simulink model "DYNctl_ver4_etud_lineaire"  (R2014b)
settings: Solver=ode45  StartTime=0.0  StopTime=tfin  FixedStep=0.001  RelTol=1e-09
values from neighbouring files (symbols this model uses):
  A = sym('A', [13 13])    [MatlabProjet.m]    (also in bancessai_ini.m = double(subs(A)); equilibre.m = double(subs(A)))
  B = sym('B', [13 3])    [MatlabProjet.m]    (also in bancessai_ini.m = double(subs(B)); equilibre.m = double(subs(B)))
  C = sym('B', [7 13])    [MatlabProjet.m]    (also in bancessai_ini.m = double(subs(C)); equilibre.m = double(subs(C)); interpolationGenerique.m = phi\y)
  D = zeros(7, 3)    [MatlabProjet.m]    (also in bancessai_ini.m = double(subs(D)); equilibre.m = double(subs(D)); matrices_syms.m)
  v_sx_eq = 0    [MatlabEquilibre.m]
  v_sy_eq = 0    [MatlabEquilibre.m]
  Va_eq = R_bobine * Ia_eq    [MatlabEquilibre.m]    (also in bancessai_ini.m = Ia_eq*R_bobine; equilibre.m = Ia_eq*R_bobine)
  xs_eq = xs    (= 0)    [equilibre.m]
  ys_eq = ys    (= 0)    [equilibre.m]
undefined symbols (not defined in the file or in its folder): sym2poly, zD_eq, zE_eq, zF_eq
settings Model: Creator=delafontaine  LastModifiedBy=Eric
settings SolverCC: AlgebraicLoopSolver=LineSearch
settings DataIOCC: SignalLoggingSaveFormat=ModelDataLogs
settings DebuggingCC: UnderspecifiedInitializationDetection=Classic  MergeDetectMultiDrivingBlocksExec=none  SolverPrmCheckMsg=none  MultiTaskDSMMsg=warning  MultiTaskCondExecSysMsg=none  FrameProcessingCompatibilityMsg=error
settings RTWCC: IncludeERTFirstTime=on

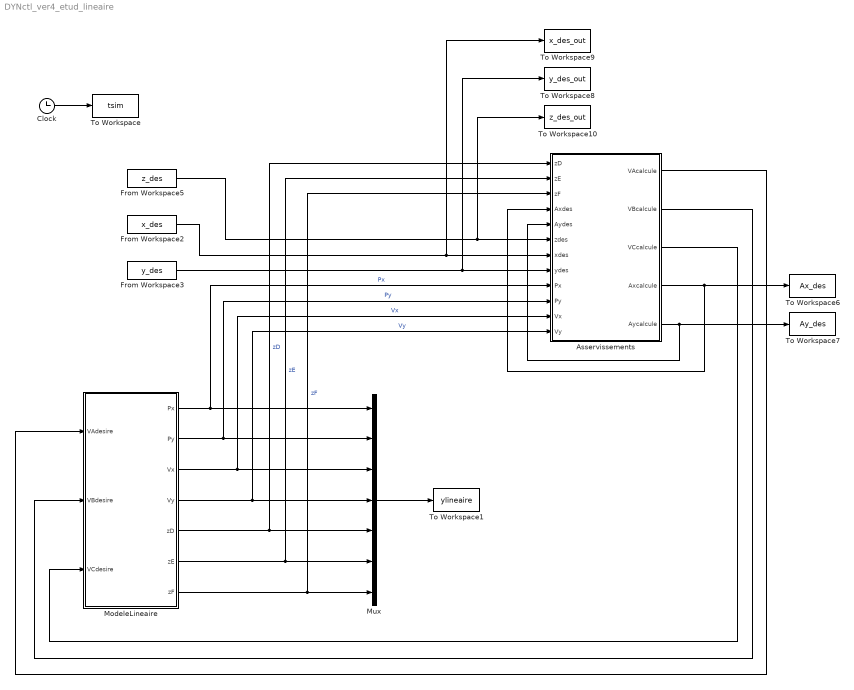
== system DYNctl_ver4_etud_lineaire ==
  Asservissements : Subsystem
      mask help: Simulink:masks:GenSFuncDesc_MD
      mask Help: eval('feval(''rtwprivate'',''rtwhelpview'',''rtw_sfcn_block'')');
  Clock : Clock
  From Workspace2 : FromWorkspace  VariableName=x_des  SampleTime=0  Interpolate=off  OutputAfterFinalValue=Holding final value
  From Workspace3 : FromWorkspace  VariableName=y_des  SampleTime=0  Interpolate=off  OutputAfterFinalValue=Holding final value
  From Workspace5 : FromWorkspace  VariableName=z_des  SampleTime=0  Interpolate=off  OutputAfterFinalValue=Holding final value
  ModeleLineaire : Subsystem
      mask help: Simulink:masks:GenSFuncDesc_MD
      mask Help: eval('feval(''rtwprivate'',''rtwhelpview'',''rtw_sfcn_block'')');
  Mux : Mux  Inputs=7
  To Workspace : ToWorkspace  VariableName=tsim  SampleTime=-1
  To Workspace1 : ToWorkspace  VariableName=ylineaire  SampleTime=-1
  To Workspace10 : ToWorkspace  VariableName=z_des_out  SampleTime=-1
  To Workspace6 : ToWorkspace  VariableName=Ax_des  SampleTime=-1
  To Workspace7 : ToWorkspace  VariableName=Ay_des  SampleTime=-1
  To Workspace8 : ToWorkspace  VariableName=y_des_out  SampleTime=-1
  To Workspace9 : ToWorkspace  VariableName=x_des_out  SampleTime=-1
  wires:
  Clock/1 -> To Workspace/1
  From Workspace5/1 -> To Workspace10/1, Asservissements/6(zdes)
  From Workspace3/1 -> Asservissements/8(ydes), To Workspace8/1
  From Workspace2/1 -> Asservissements/7(xdes), To Workspace9/1
  Asservissements/4(Axcalcule) -> Asservissements/4(Axdes), To Workspace6/1
  Asservissements/5(Aycalcule) -> Asservissements/5(Aydes), To Workspace7/1
  Asservissements/1(VAcalcule) -> ModeleLineaire/1(VAdesire)
  Asservissements/2(VBcalcule) -> ModeleLineaire/2(VBdesire)
  Asservissements/3(VCcalcule) -> ModeleLineaire/3(VCdesire)
  ModeleLineaire/5(zD) -> Mux/5, Asservissements/1(zD)  "zD"
  ModeleLineaire/6(zE) -> Mux/6, Asservissements/2(zE)  "zE"
  ModeleLineaire/7(zF) -> Mux/7, Asservissements/3(zF)  "zF"
  ModeleLineaire/1(Px) -> Mux/1, Asservissements/9(Px)  "Px"
  ModeleLineaire/2(Py) -> Asservissements/10(Py), Mux/2  "Py"
  ModeleLineaire/3(Vx) -> Asservissements/11(Vx), Mux/3  "Vx"
  ModeleLineaire/4(Vy) -> Asservissements/12(Vy), Mux/4  "Vy"
  Mux/1 -> To Workspace1/1

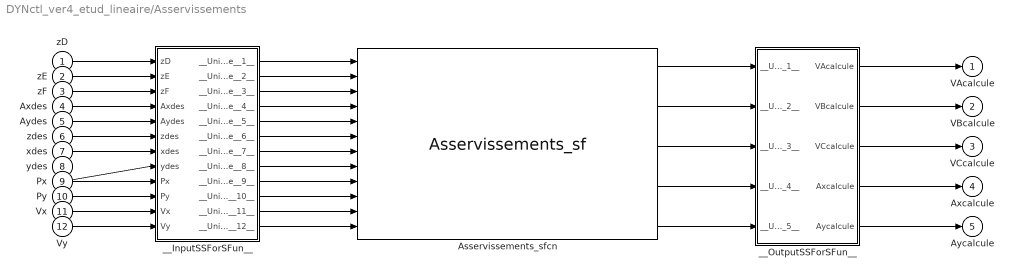
== system DYNctl_ver4_etud_lineaire/Asservissements ==
  zD : Inport
  zE : Inport  Port=2
  zF : Inport  Port=3
  Axdes : Inport  Port=4
  Aydes : Inport  Port=5
  zdes : Inport  Port=6
  xdes : Inport  Port=7
  ydes : Inport  Port=8
  Px : Inport  Port=9
  Py : Inport  Port=10
  Vx : Inport  Port=11
  Vy : Inport  Port=12
  Asservissements_sfcn : S-Function  FunctionName=Asservissements_sf  SFunctionModules=""  EnableBusSupport=off  mask{rtw_sf_name=Asservissements_sf, showVar=off}
      mask prompts: rtw_sf_name "Simulink:masks:GenSFuncName_MP"; showVar "Simulink:masks:GenSFuncShowModuleList_MP"
      mask help: Simulink:masks:GenSFuncDesc_MD
      mask init:
      | displist = '';
      | if ~strcmp(get_param(gcb, 'FunctionName'), rtw_sf_name);
      |   set_param(gcb, 'FunctionName', rtw_sf_name);
      | end
      | % Check if we are generating code
      | rtw_mode = false;
      | if strcmpi(get_param(bdroot(gcb),'SimulationStatus'),'Initializing')
      | 	rtw_mode = strcmpi(get_param(bdroot(gcb),'BuildingRTWCode'),'on') && ...
      | 		~strcmpi(get_param(bdroot(gcb),'TargetStyle'),'SimulationTarget');
      | end
      | if showVar || rtw_mode
      | 	if exist('rtwsfunc') == 2 | exist('rtwsfunc') == 6
      | 		tmplist = rtwsfunc(rtw_sf_name,gcb);
      | 		tmplist = DAStudio.message('Simulink:masks:GenSFuncListOfModules_IC', tmplist);
      | 	elseif showVar
      | 		tmplist1 = DAStudio.message('Simulink:masks:GenSFuncListOfModules_IC', '');
      |         tmplist2 = DAStudio.message('Simulink:masks:GenSFuncNotLicensed_IC');
      |         tmplist = [tmplist1 tmplist2];
      |  	end
      | end
      | if showVar
      |   displist = tmplist;
      | end
      settings: CopyFcn=|
      | if ~strcmp(get_param(gcb,'Linkstatus'),'none') && ...
      | ~strcmp(get_param(gcb,'Linkstatus'),'implicit')
      |   set_param(gcb,'LinkStatus','none');
      | end
      mask Help: eval('feval(''rtwprivate'',''rtwhelpview'',''rtw_sfcn_block'')');
      mask Display:
      | port_label('input',1,'zD');
      | port_label('input',2,'zE');
      | port_label('input',3,'zF');
      | port_label('input',4,'Axdes');
      | port_label('input',5,'Aydes');
      | port_label('input',6,'zdes');
      | port_label('input',7,'xdes');
      | port_label('input',8,'ydes');
      | port_label('input',9,'Px');
      | port_label('input',10,'Py');
      | port_label('input',11,'Vx');
      | port_label('input',12,'Vy');
      | port_label('output',1,'VAcalcule');
      | port_label('output',2,'VBcalcule');
      | port_label('output',3,'VCcalcule');
      | port_label('output',4,'Axcalcule');
      | port_label('output',5,'Aycalcule');
  __InputSSForSFun__ : Subsystem
  __OutputSSForSFun__ : Subsystem
  VAcalcule : Outport
  VBcalcule : Outport  Port=2
  VCcalcule : Outport  Port=3
  Axcalcule : Outport  Port=4
  Aycalcule : Outport  Port=5
  wires:
  zD/1 -> __InputSSForSFun__/1(zD)
  zE/1 -> __InputSSForSFun__/2(zE)
  zF/1 -> __InputSSForSFun__/3(zF)
  Axdes/1 -> __InputSSForSFun__/4(Axdes)
  Aydes/1 -> __InputSSForSFun__/5(Aydes)
  zdes/1 -> __InputSSForSFun__/6(zdes)
  xdes/1 -> __InputSSForSFun__/7(xdes)
  ydes/1 -> __InputSSForSFun__/8(ydes)
  Px/1 -> __InputSSForSFun__/9(Px)
  Py/1 -> __InputSSForSFun__/10(Py)
  Vx/1 -> __InputSSForSFun__/11(Vx)
  Vy/1 -> __InputSSForSFun__/12(Vy)
  __InputSSForSFun__/1(__UniqueOutportName__1__) -> Asservissements_sfcn/1
  __InputSSForSFun__/2(__UniqueOutportName__2__) -> Asservissements_sfcn/2
  __InputSSForSFun__/3(__UniqueOutportName__3__) -> Asservissements_sfcn/3
  __InputSSForSFun__/4(__UniqueOutportName__4__) -> Asservissements_sfcn/4
  __InputSSForSFun__/5(__UniqueOutportName__5__) -> Asservissements_sfcn/5
  __InputSSForSFun__/6(__UniqueOutportName__6__) -> Asservissements_sfcn/6
  __InputSSForSFun__/7(__UniqueOutportName__7__) -> Asservissements_sfcn/7
  __InputSSForSFun__/8(__UniqueOutportName__8__) -> Asservissements_sfcn/8
  __InputSSForSFun__/9(__UniqueOutportName__9__) -> Asservissements_sfcn/9
  __InputSSForSFun__/10(__UniqueOutportName__10__) -> Asservissements_sfcn/10
  __InputSSForSFun__/11(__UniqueOutportName__11__) -> Asservissements_sfcn/11
  __InputSSForSFun__/12(__UniqueOutportName__12__) -> Asservissements_sfcn/12
  Asservissements_sfcn/1 -> __OutputSSForSFun__/1(__UniqueInportName__1__)
  Asservissements_sfcn/2 -> __OutputSSForSFun__/2(__UniqueInportName__2__)
  Asservissements_sfcn/3 -> __OutputSSForSFun__/3(__UniqueInportName__3__)
  Asservissements_sfcn/4 -> __OutputSSForSFun__/4(__UniqueInportName__4__)
  Asservissements_sfcn/5 -> __OutputSSForSFun__/5(__UniqueInportName__5__)
  __OutputSSForSFun__/1(VAcalcule) -> VAcalcule/1
  __OutputSSForSFun__/2(VBcalcule) -> VBcalcule/1
  __OutputSSForSFun__/3(VCcalcule) -> VCcalcule/1
  __OutputSSForSFun__/4(Axcalcule) -> Axcalcule/1
  __OutputSSForSFun__/5(Aycalcule) -> Aycalcule/1

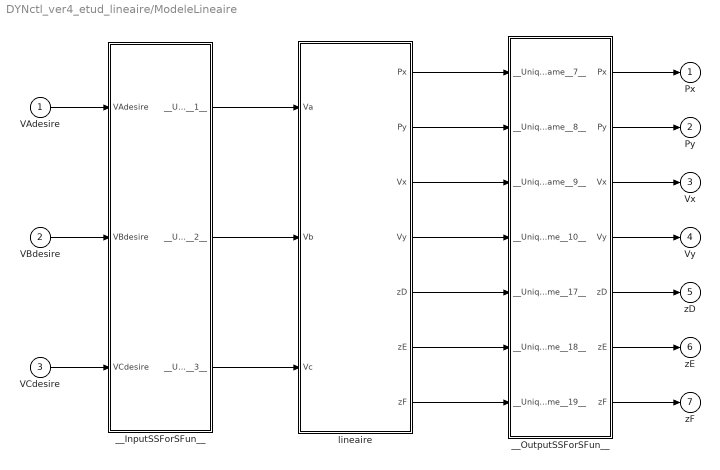
== system DYNctl_ver4_etud_lineaire/ModeleLineaire ==
  VAdesire : Inport
  VBdesire : Inport  Port=2
  VCdesire : Inport  Port=3
  __InputSSForSFun__ : Subsystem
  __OutputSSForSFun__ : Subsystem
  lineaire : Subsystem
  Px : Outport
  Py : Outport  Port=2
  Vx : Outport  Port=3
  Vy : Outport  Port=4
  zD : Outport  Port=5
  zE : Outport  Port=6
  zF : Outport  Port=7
  wires:
  VAdesire/1 -> __InputSSForSFun__/1(VAdesire)
  VBdesire/1 -> __InputSSForSFun__/2(VBdesire)
  VCdesire/1 -> __InputSSForSFun__/3(VCdesire)
  __InputSSForSFun__/1(__UniqueOutportName__1__) -> lineaire/1(Va)
  __InputSSForSFun__/2(__UniqueOutportName__2__) -> lineaire/2(Vb)
  __InputSSForSFun__/3(__UniqueOutportName__3__) -> lineaire/3(Vc)
  lineaire/5(zD) -> __OutputSSForSFun__/5(__UniqueInportName__17__)
  lineaire/6(zE) -> __OutputSSForSFun__/6(__UniqueInportName__18__)
  lineaire/7(zF) -> __OutputSSForSFun__/7(__UniqueInportName__19__)
  lineaire/1(Px) -> __OutputSSForSFun__/1(__UniqueInportName__7__)
  lineaire/2(Py) -> __OutputSSForSFun__/2(__UniqueInportName__8__)
  lineaire/3(Vx) -> __OutputSSForSFun__/3(__UniqueInportName__9__)
  lineaire/4(Vy) -> __OutputSSForSFun__/4(__UniqueInportName__10__)
  __OutputSSForSFun__/1(Px) -> Px/1
  __OutputSSForSFun__/2(Py) -> Py/1
  __OutputSSForSFun__/3(Vx) -> Vx/1
  __OutputSSForSFun__/4(Vy) -> Vy/1
  __OutputSSForSFun__/5(zD) -> zD/1
  __OutputSSForSFun__/6(zE) -> zE/1
  __OutputSSForSFun__/7(zF) -> zF/1

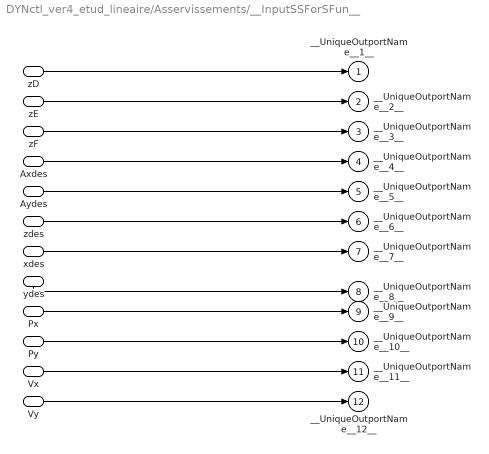
== system DYNctl_ver4_etud_lineaire/Asservissements/__InputSSForSFun__ ==
  zD : Inport
  zE : Inport  Port=2
  zF : Inport  Port=3
  Axdes : Inport  Port=4
  Aydes : Inport  Port=5
  zdes : Inport  Port=6
  xdes : Inport  Port=7
  ydes : Inport  Port=8
  Px : Inport  Port=9
  Py : Inport  Port=10
  Vx : Inport  Port=11
  Vy : Inport  Port=12
  __UniqueOutportName__1__ : Outport
  __UniqueOutportName__2__ : Outport  Port=2
  __UniqueOutportName__3__ : Outport  Port=3
  __UniqueOutportName__4__ : Outport  Port=4
  __UniqueOutportName__5__ : Outport  Port=5
  __UniqueOutportName__6__ : Outport  Port=6
  __UniqueOutportName__7__ : Outport  Port=7
  __UniqueOutportName__8__ : Outport  Port=8
  __UniqueOutportName__9__ : Outport  Port=9
  __UniqueOutportName__10__ : Outport  Port=10
  __UniqueOutportName__11__ : Outport  Port=11
  __UniqueOutportName__12__ : Outport  Port=12
  wires:
  zD/1 -> __UniqueOutportName__1__/1
  zE/1 -> __UniqueOutportName__2__/1
  zF/1 -> __UniqueOutportName__3__/1
  Axdes/1 -> __UniqueOutportName__4__/1
  Aydes/1 -> __UniqueOutportName__5__/1
  zdes/1 -> __UniqueOutportName__6__/1
  xdes/1 -> __UniqueOutportName__7__/1
  ydes/1 -> __UniqueOutportName__8__/1
  Px/1 -> __UniqueOutportName__9__/1
  Py/1 -> __UniqueOutportName__10__/1
  Vx/1 -> __UniqueOutportName__11__/1
  Vy/1 -> __UniqueOutportName__12__/1

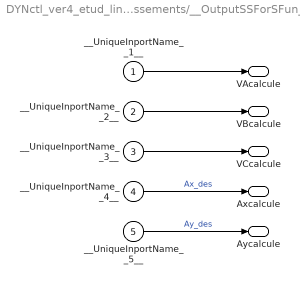
== system DYNctl_ver4_etud_lineaire/Asservissements/__OutputSSForSFun__ ==
  __UniqueInportName__1__ : Inport
  __UniqueInportName__2__ : Inport  Port=2
  __UniqueInportName__3__ : Inport  Port=3
  __UniqueInportName__4__ : Inport  Port=4
  __UniqueInportName__5__ : Inport  Port=5
  VAcalcule : Outport
  VBcalcule : Outport  Port=2
  VCcalcule : Outport  Port=3
  Axcalcule : Outport  Port=4
  Aycalcule : Outport  Port=5
  wires:
  __UniqueInportName__1__/1 -> VAcalcule/1
  __UniqueInportName__2__/1 -> VBcalcule/1
  __UniqueInportName__3__/1 -> VCcalcule/1
  __UniqueInportName__4__/1 -> Axcalcule/1  "Ax_des"
  __UniqueInportName__5__/1 -> Aycalcule/1  "Ay_des"

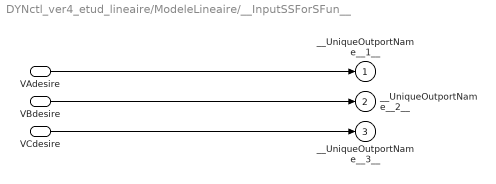
== system DYNctl_ver4_etud_lineaire/ModeleLineaire/__InputSSForSFun__ ==
  VAdesire : Inport
  VBdesire : Inport  Port=2
  VCdesire : Inport  Port=3
  __UniqueOutportName__1__ : Outport
  __UniqueOutportName__2__ : Outport  Port=2
  __UniqueOutportName__3__ : Outport  Port=3
  wires:
  VAdesire/1 -> __UniqueOutportName__1__/1
  VBdesire/1 -> __UniqueOutportName__2__/1
  VCdesire/1 -> __UniqueOutportName__3__/1

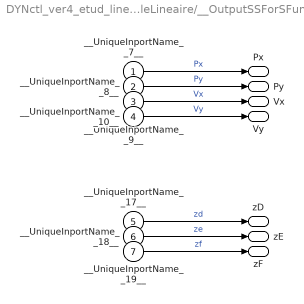
== system DYNctl_ver4_etud_lineaire/ModeleLineaire/__OutputSSForSFun__ ==
  __UniqueInportName__7__ : Inport
  __UniqueInportName__8__ : Inport  Port=2
  __UniqueInportName__9__ : Inport  Port=3
  __UniqueInportName__10__ : Inport  Port=4
  __UniqueInportName__17__ : Inport  Port=5
  __UniqueInportName__18__ : Inport  Port=6
  __UniqueInportName__19__ : Inport  Port=7
  Px : Outport
  Py : Outport  Port=2
  Vx : Outport  Port=3
  Vy : Outport  Port=4
  zD : Outport  Port=5
  zE : Outport  Port=6
  zF : Outport  Port=7
  wires:
  __UniqueInportName__7__/1 -> Px/1  "Px"
  __UniqueInportName__8__/1 -> Py/1  "Py"
  __UniqueInportName__9__/1 -> Vx/1  "Vx"
  __UniqueInportName__10__/1 -> Vy/1  "Vy"
  __UniqueInportName__17__/1 -> zD/1  "zd"
  __UniqueInportName__18__/1 -> zE/1  "ze"
  __UniqueInportName__19__/1 -> zF/1  "zf"

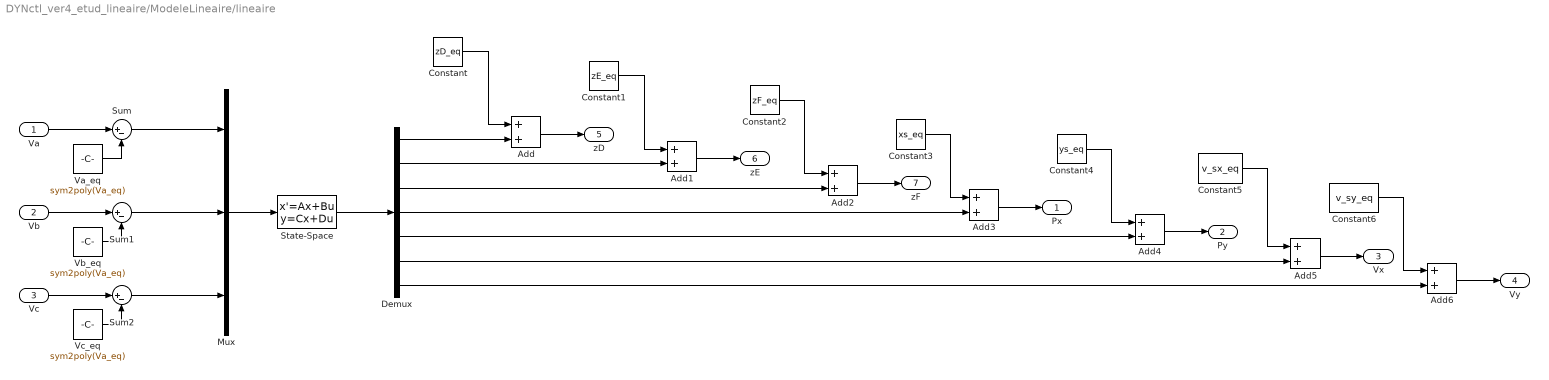
== system DYNctl_ver4_etud_lineaire/ModeleLineaire/lineaire ==
  Va : Inport
  Vb : Inport  Port=2
  Vc : Inport  Port=3
  Add{,1..6} (7 alike) : Sum
  Constant : Constant  Value=zD_eq
  Constant1 : Constant  Value=zE_eq
  Constant2 : Constant  Value=zF_eq
  Constant3 : Constant  Value=xs_eq
  Constant4 : Constant  Value=ys_eq
  Constant5 : Constant  Value=v_sx_eq
  Constant6 : Constant  Value=v_sy_eq
  Demux : Demux  Outputs=7
  Mux : Mux  Inputs=3
  State-Space : StateSpace  A=A  B=B  C=C  D=D  X0=0
  Sum : Sum  Inputs=|+-
  Sum1 : Sum  Inputs=|+-
  Sum2 : Sum  Inputs=|+-
  Va_eq : Constant  Value=sym2poly(Va_eq)
  Vb_eq : Constant  Value=sym2poly(Va_eq)
  Vc_eq : Constant  Value=sym2poly(Va_eq)
  Px : Outport
  Py : Outport  Port=2
  Vx : Outport  Port=3
  Vy : Outport  Port=4
  zD : Outport  Port=5
  zE : Outport  Port=6
  zF : Outport  Port=7
  wires:
  Va/1 -> Sum/1
  Mux/1 -> State-Space/1
  Vb/1 -> Sum1/1
  Vc/1 -> Sum2/1
  Sum1/1 -> Mux/2
  Sum/1 -> Mux/1
  Sum2/1 -> Mux/3
  Va_eq/1 -> Sum/2
  Vb_eq/1 -> Sum1/2
  Vc_eq/1 -> Sum2/2
  State-Space/1 -> Demux/1
  Demux/1 -> Add/2
  Add/1 -> zD/1
  Constant/1 -> Add/1
  Demux/2 -> Add1/2
  Add1/1 -> zE/1
  Constant1/1 -> Add1/1
  Demux/3 -> Add2/2
  Add2/1 -> zF/1
  Constant2/1 -> Add2/1
  Demux/4 -> Add3/2
  Add3/1 -> Px/1
  Constant3/1 -> Add3/1
  Demux/5 -> Add4/2
  Add4/1 -> Py/1
  Constant4/1 -> Add4/1
  Demux/6 -> Add5/2
  Add5/1 -> Vx/1
  Constant5/1 -> Add5/1
  Demux/7 -> Add6/2
  Add6/1 -> Vy/1
  Constant6/1 -> Add6/1
